simulink model "Modelsim"  (R2024a)
settings: Solver=VariableStepAuto  StartTime=0.0  StopTime=60  RelTol=1e-3
PreLoadFcn:
  | maxNumErrs = 100;
  | maxNumBits = 1e6;
  | EbNo = 4;
undefined symbols (not defined in the file): designMultirateFIR, SimPara
libraries: commchan3 x3, simulink x2, commcnvcod2 x2, dspvision x2, commdigbbndpm3 x2, commfilt2 x2, dspindex x2, matrix_library x2, dspsnks4 x1, commsink2 x1, dspmlti4 x1, commutil2 x1
settings Model: MinMaxOverflowLogging=MinMaxAndOverflow  SimulationMode=accelerator  Creator=The MathWorks, Inc.  LastModifiedBy=fiona
settings SolverCC: AlgebraicLoopSolver=TrustRegion
settings DataIOCC: LimitDataPoints=on  SaveFormat=Array  SignalLogging=off  SaveTime=off  ReturnWorkspaceOutputs=off
settings OptimizationCC: DefaultParameterBehavior=Inlined  ReuseModelBlockBuffer=off  ExpressionDepthLimit=2147483647  LocalBlockOutputs=off  InitFltsAndDblsToZero=on  LifeSpan=1  EfficientTunableParamExpr=on
settings DebuggingCC: SaveWithParameterizedLinksMsg=none  SignalResolutionControl=TryResolveAllWithWarning  SolverPrmCheckMsg=warning  MultiTaskDSMMsg=warning  MultiTaskCondExecSysMsg=none  UnconnectedInputMsg=warning  UnconnectedOutputMsg=warning  UnconnectedLineMsg=warning  StateNameClashWarn=warning  SFUnexpectedBacktrackingDiag=warning  SFNoUnconditionalDefaultTransitionDiag=warning  SFExecutionAtInitializationDiag=none  ArithmeticOperatorsInVariantConditions=warning
settings HardwareCC: ProdBitPerInt=16  ProdBitPerPointer=32  ProdBitPerSizeT=16  ProdBitPerPtrDiffT=16  ProdLargestAtomicFloat=None  ProdIntDivRoundTo=Floor  ProdWordSize=16  ProdHWDeviceType=16-bit Generic  TargetBitPerPointer=64  TargetBitPerSizeT=64  TargetBitPerPtrDiffT=64  TargetLongLongMode=on  TargetIntDivRoundTo=Zero  TargetEndianess=LittleEndian  TargetWordSize=64  TargetHWDeviceType=MATLAB Host  ProdEqTarget=off
settings ModelReferenceCC: EnableRefExpFcnMdlSchedulingChecks=on  PropagateSignalLabelsOutOfModel=off
settings SFSimCC: SimUseLocalCustomCode=off  MATLABDynamicMemAlloc=off  CustomCodeUndefinedFunction=UseInterfaceOnly
settings RTWCC: Description=Real-Time Workshop Embedded Coder (no auto configuration)  SystemTargetFile=ert.tlc  TemplateMakefile=ert_default_tmf  GenerateReport=on  RetainRTWFile=on  RTWUseLocalCustomCode=off  IncludeHyperlinkInReport=on  LaunchReport=on  GPUComputeCapability=3.5
settings CodeAppCC: CustomSymbolStrType=$N$R$M  StateflowObjectComments=on  InternalIdentifier=Classic
settings ERTTargetCC: TargetFcnLib=ansi_tfl_tmw.mat  MultiwordLength=2048  GenerateSampleERTMain=on  SupportAbsoluteTime=off  MatFileLogging=on  InlinedParameterPlacement=NonHierarchical  ERTCustomFileTemplate=example_file_process.tlc  ConvertIfToSwitch=off  SuppressUnreachableDefaultCases=off
settings ConfigComp: CovMetricSettings=dw  CovSaveCumulativeToWorkspaceVar=on  CovSaveSingleToWorkspaceVar=on  CovExternalEMLEnable=off

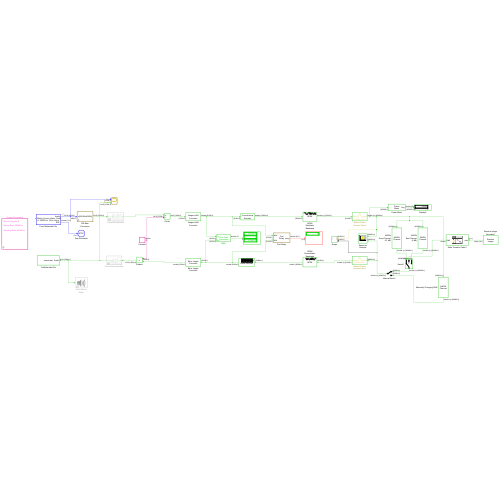
[thumbnail: Simulink's stored preview of the top-level diagram]
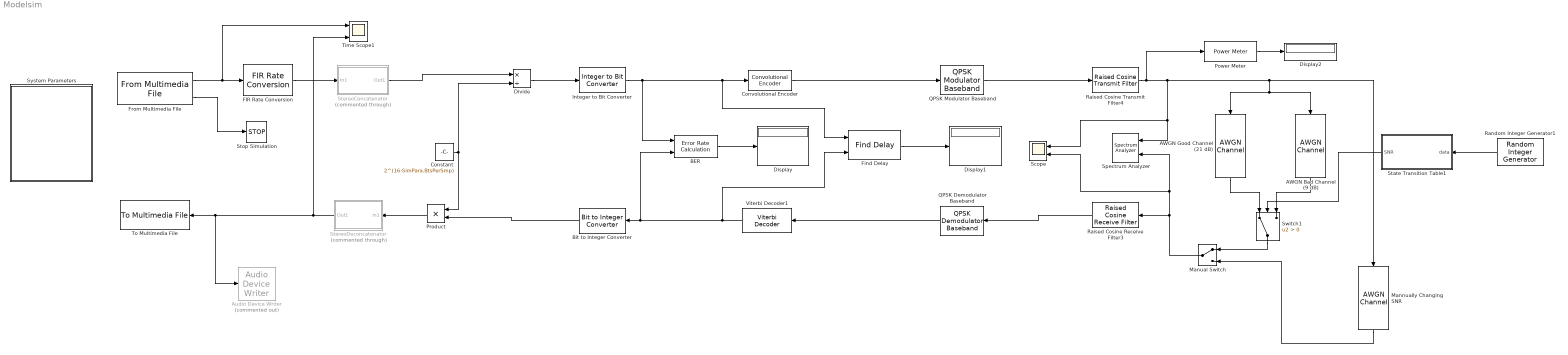
== system Modelsim ==
  AWGN Bad Channel (9 dB) : commchan3/AWGN Channel  LegacyMode=on  NoiseMethod="Signal to noise ratio  (SNR)"  noiseMode="Signal to noise ratio  (SNR)"  EbNo=10  EsNo=10  SNR=9  BitsPerSymbol=1  SignalPower=1  SamplesPerSymbol=1  SymbolPeriod=1  VarianceSource=Parameter  Variance=1  RandomStream=Global stream  Seed=67  SimulateUsing=Code generation
  AWGN Good Channel (21 dB) : commchan3/AWGN Channel  LegacyMode=on  NoiseMethod="Signal to noise ratio  (SNR)"  noiseMode="Signal to noise ratio  (SNR)"  EbNo=10  EsNo=10  SNR=21  BitsPerSymbol=1  SignalPower=1  SamplesPerSymbol=1  SymbolPeriod=1  VarianceSource=Parameter  Variance=1  RandomStream=Global stream  Seed=67  SimulateUsing=Code generation
  Audio Device Writer : dspsnks4/Audio Device Writer  Commented=on  Driver=DirectSound  Device=Default  InheritSampleRate=on  SampleRate=44100  BitDepth=16-bit integer  BufferSize=4096  NumBuffers=10  DefaultOutputChannelMapping=on  OutputChannelMapping=1:2  OutputNumUnderrunSamples=off  DriverIdx=1  DeviceWarnFlag=''
  BER : commsink2/Error Rate Calculation  N=20  st_delay=0  cp_mode=Entire frame  subframe=[]  PMode=Port  WsName=ErrorVec  RsMode2=off  stop=off  numErr=100  maxBits=1e7
  Bit to Integer Converter : simulink/Logic and Bit Operations/Bit to Integer Converter  nbits=SimPara.BtsPerSmp  bitOrder=MSB first  signedOutputValues=Signed  outDtype=Inherit via internal rule  outDtypeSigned=Inherit via internal rule
  Constant : Constant  Value=2^(16-SimPara.BtsPerSmp)
  Convolutional Encoder : commcnvcod2/Convolutional Encoder  trellis=poly2trellis(3, [7 5])  opMode=Continuous  DelayedResetAction=off  hasIniStPort=off  hasFinStPort=off  usePuncVector=off  punctureVector=[1; 1; 0; 1; 0; 1]  reset=Unused parameter value
  Display : Display
  Display1 : Display
  Display2 : Display
  Divide : Product  Inputs=*/  OutDataTypeStr=Inherit: Same as first input
  FIR Rate Conversion : dspmlti4/FIR Rate Conversion  FilterSource=Auto  L=SimPara.SmpRte  h=designMultirateFIR(3,2)  M=SimPara.SrcRte  FilterObject=FRC  rateMode=Allow multirate processing  AllowArbitraryInputLength=on  roundingMode=Floor  overflowMode=off  firstCoeffDataTypeStr=Inherit: Same word length as input  firstCoeffMin=[]  firstCoeffMax=[]  firstCoeffLastDataTypeStr=Inherit: Same word length as input  outputMin=[]  outputMax=[]
  Find Delay : commutil2/Find Delay  corrLength=1000  chgSigOP=off  stopUpdate=off  numConstDelay=3
  From Multimedia File : dspvision/From Multimedia File  inputFilename=C:\UBC\ELEC391\SoundFiles\Mono_16bit_22kHz_Uncom_60sec_PinkPanther.wav  readRange=[1 Inf]  loop=on  numPlays=1  outputStreams=Audio only  videoDataType=single  audioDataType=int16  inheritSampleTime=on  userDefinedSampleTime=1/30  noAudioOutput=off  isIntensityVideo=off  fourcc=RGB  colorVideoFormat=Separate color signals  outputEOF=on  dataOrg=Column-major  audioFrameSize=1024  computeAudioFrameSize=off  outSamplingMode=Sample based
      settings: LibrarySourceBlock=audiosources/From Multimedia File
  Integer to Bit Converter : simulink/Logic and Bit Operations/Integer to Bit Converter  nbits=SimPara.BtsPerSmp  signedInputValues=Signed  bitOrder=MSB first  outDtype=double
  Mannually Changing SNR : commchan3/AWGN Channel  LegacyMode=off  NoiseMethod="Signal to noise ratio  (SNR)"  noiseMode="Signal to noise ratio  (SNR)"  EbNo=10  EsNo=10  SNR=10  BitsPerSymbol=1  SignalPower=1  SamplesPerSymbol=1  SymbolPeriod=1  VarianceSource=Parameter  Variance=1  RandomStream=Global stream  Seed=67  SimulateUsing=Code generation
  Manual Switch : ManualSwitch
  Power Meter : dspstat3/Power Meter  Measurement=Average power  ReferenceLoad=1  OutputPowerUnits=Watts  WindowLength=256  OverlapLength=255  AllowArbitraryInputLength=off  ComputeCCDF=off  PowerRange=50  PowerResolution=0.1  CCDFOutput=Relative power (dB above average power)  ProbabilityVector=[ 10; 1; 0.1; 0.01; 0.001; 0.0001 ]  RelativePowerVector=[ 0; 3; 6; 9; 12 ]  ResetPort=off  SimulateUsing=Interpreted execution
  Product : Product  OutDataTypeStr=int16
  QPSK Demodulator Baseband : commdigbbndpm3/QPSK Demodulator Baseband  OutType=Bit  DecType=Hard decision  VarSource=Dialog  Variance=1  Dec=Binary  Ph=pi/4  outDtype1=Inherit via internal rule  outDtype2=Inherit via internal rule  derotateFactorWordLen=16  derotateFactorDataTypeStr=Inherit: Same word length as input  derotateFactorLastDataTypeStr=Inherit: Same word length as input
  QPSK Modulator Baseband : commdigbbndpm3/QPSK Modulator Baseband  InType=Bit  Enc=Binary  Ph=pi/4  outDtype=double  outWordLen=16  outUDDataType=sfix(16)  outFracLenMode=Best precision  outFracLen=15  outDataTypeStr=double  outLastDataTypeStr=double
  Raised Cosine Receive Filter3 : commfilt2/Raised Cosine Receive Filter  filtType=Square root  R=0.8  filtSpan=4  N=5  downFactor=5  downOffset=0  filterGain=1  InputProcessing=Columns as channels (frame based)  RateOptions=Enforce single-rate processing  framing=Mute  checkCoeff=on  variableName=rcRxFilt3  currentFiltSpan=10  D=5  inputOffset=0  sampMode=Mute  saveAsFlag=0  rateMode=Downsampling  checkGain=Normalized  launchFVT=on  roundingMode=Floor  overflowMode=off  coeffDataTypeStr=Inherit: Same word length as input  coeffMin=[]  coeffMax=[]  coeffLastDataTypeStr=Inherit: Same word length as input  accumDataTypeStr=Inherit: Same as product output  accumLastDataTypeStr=Inherit: Same as product output  outputDataTypeStr=Inherit: Same as accumulator  outputMin=[]  outputMax=[]  outputLastDataTypeStr=Inherit: Same as accumulator
      settings: LibrarySourceBlock=|
      | commhdlfilt/Raised Cosine
      | Receive Filter
  Raised Cosine Transmit Filter4 : commfilt2/Raised Cosine Transmit Filter  filtType=Square root  R=0.8  filtSpan=4  N=5  filterGain=1  InputProcessing=Columns as channels (frame based)  RateOptions=Enforce single-rate processing  framing=Mute  checkCoeff=on  variableName=rcTxFilt4  checkGain=Normalized  sampMode=Mute  saveAsFlag=0  currentFiltSpan=10  D=5  launchFVT=on  roundingMode=Floor  overflowMode=off  coeffDataTypeStr=Inherit: Same word length as input  coeffMin=[]  coeffMax=[]  coeffLastDataTypeStr=Inherit: Same word length as input  outputDataTypeStr=Inherit: Same as accumulator  outputMin=[]  outputMax=[]  outputLastDataTypeStr=Inherit: Same as accumulator
      settings: LibrarySourceBlock=|
      | commhdlfilt/Raised Cosine
      | Transmit Filter
  Random Integer Generator1 : commrandsrc3/Random Integer Generator  SetSize=100  SeedSource=Auto  Seed=0  SampleTime=0.0256  SamplesPerFrame=1  OutputDataType=single  SimulateUsing=Interpreted execution
  Scope : Scope  NumInputPorts=2
  Spectrum Analyzer : SpectrumAnalyzer  NumInputPorts=2  WindowPosition=[1.000000,49.000000,1504.000000,932.000000,]  ScopeFrameLocation=window  FrequencySpan=Start and stop frequencies  StartFrequency=0  StopFrequency=600000  YLimits=[-142.8961798129679,30.326241209565428]  ShowLegend=on  SelectedToolstripTab=spectrumAnalyzerToolstrip.channelMeasurementsTab  MeasurementChannel=2
  State Transition Table1 : State Transition Table  TreatAsAtomicUnit=on
  StereoConcatenator : Subsystem  Commented=through
  StereoDeconcatenator : Subsystem  Commented=through
  Stop Simulation : Stop
  Switch1 : Switch  Criteria=u2 > Threshold  SaturateOnIntegerOverflow=off  InputSameDT=off
  System Parameters : Subsystem  mask{BtsPerSmp=8, SrcRte=22050, SmpRte=40000}
      mask prompts: BtsPerSmp "BitsPerSample"; SrcRte "Source Rate (Hz)"; SmpRte "Sampling Rate (Hz)"
      mask init:
      | info.BtsPerSmp = BtsPerSmp;
      | info.SmpRte = SmpRte;
      | info.SrcRte = SrcRte;
      | 
      | assignin('base', 'SimPara', info);
      mask DialogControl SimVar Prompt: SimVariables
      mask Display:
      | text( ...
      |     10, 140, ...
      |     [ ...
      |     '\n\nBits Per Sample: ', num2str(BtsPerSmp), ...
      |     '\n\nSource Rate: ', num2str(SrcRte) ' Hz', ...
      |     '\n\nSampling Rate: ', num2str(SmpRte) ' Hz'], ...
      |     'horizontalAlignment', 'left' ...
      |     )
  Time Scope1 : Scope  NumInputPorts=3
  To Multimedia File : dspvision/To Multimedia File  outputFilename=C:\UBC\ELEC391\output.wav  streamSelection=Audio only  videoCompressor=None (uncompressed)  audioCompressor=None (uncompressed)  imagePorts=One multidimensional signal  fileType=WAV  audioDatatype=Determine from input data type  fourcc=RGB  audioBitRate=128  audioQuality=75  videoQuality=75  mj2000CompFactor=10
      settings: LibrarySourceBlock=audiosinks/To Multimedia File
  Viterbi Decoder1 : commcnvcod2/Viterbi Decoder  trellis=poly2trellis(3, [7 5])  isPunctured=off  punctureVector=[1; 1; 0; 1; 0; 1]  erasures=off  dectype=Hard decision  nsdecb=3  runSigValErrCheck=off  tbdepth=16  opmode=Continuous  reset=off  delayedResetAction=off  smWordLength=16  outDataType=double
  wires:
  BER/1 -> Display/1
  From Multimedia File/1 -> Time Scope1/1, FIR Rate Conversion/1
  FIR Rate Conversion/1 -> StereoConcatenator/1(In1)
  Divide/1 -> Integer to Bit Converter/1
  StereoDeconcatenator/1(Out1) -> Audio Device Writer/1, To Multimedia File/1, Time Scope1/3
  Product/1 -> StereoDeconcatenator/1(In1)
  StereoConcatenator/1(Out1) -> Divide/1
  Bit to Integer Converter/1 -> Product/2
  Constant/1 -> Product/1, Divide/2
  From Multimedia File/2 -> Stop Simulation/1
  QPSK Modulator Baseband/1 -> Raised Cosine Transmit Filter4/1
  QPSK Demodulator Baseband/1 -> Viterbi Decoder1/1
  Integer to Bit Converter/1 -> BER/1, Find Delay/1, Convolutional Encoder/1
  Raised Cosine Receive Filter3/1 -> QPSK Demodulator Baseband/1
  Convolutional Encoder/1 -> QPSK Modulator Baseband/1
  Random Integer Generator1/1 -> State Transition Table1/1(data)
  AWGN Good Channel (21 dB)/1 -> Switch1/1
  AWGN Bad Channel (9 dB)/1 -> Switch1/3
  State Transition Table1/1(SNR) -> Switch1/2
  Raised Cosine Transmit Filter4/1 -> Scope/1, Spectrum Analyzer/1, Mannually Changing SNR/1, AWGN Bad Channel (9 dB)/1, AWGN Good Channel (21 dB)/1, Power Meter/1
  Viterbi Decoder1/1 -> Find Delay/2, BER/2, Bit to Integer Converter/1
  Find Delay/1 -> Display1/1
  Power Meter/1 -> Display2/1
  Manual Switch/1 -> Scope/2, Spectrum Analyzer/2, Raised Cosine Receive Filter3/1
  Switch1/1 -> Manual Switch/1
  Mannually Changing SNR/1 -> Manual Switch/2

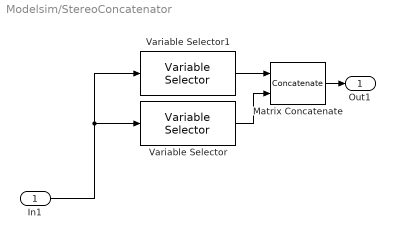
== system Modelsim/StereoConcatenator ==
  In1 : Inport
  Matrix Concatenate : Concatenate  ConcatenateDimension=2
  Variable Selector : dspindex/Variable Selector  NumInputs=1  rowsOrCols=Columns  IdxMode=Fixed  Elements=[1]  ZerOneIdxMode=One-based  errmode=Clip Index  FillMode=on  FillValues=0
  Variable Selector1 : dspindex/Variable Selector  NumInputs=1  rowsOrCols=Columns  IdxMode=Fixed  Elements=[2]  ZerOneIdxMode=One-based  errmode=Clip Index  FillMode=on  FillValues=0
  Out1 : Outport
  wires:
  Variable Selector1/1 -> Matrix Concatenate/1
  In1/1 -> Variable Selector1/1, Variable Selector/1
  Variable Selector/1 -> Matrix Concatenate/2
  Matrix Concatenate/1 -> Out1/1

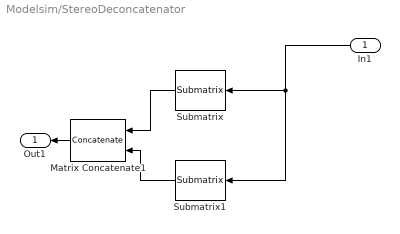
== system Modelsim/StereoDeconcatenator ==
  In1 : Inport
  Matrix Concatenate1 : Concatenate  Mode=Multidimensional array  ConcatenateDimension=2
  Submatrix : matrix_library/Submatrix  RowSpan=Range of rows  RowStartMode=First  RowStartIndex=1  RowEndMode=Offset from middle  RowEndIndex=-1  ColSpan=All columns  ColStartMode=First  ColStartIndex=1  ColEndMode=Last  ColEndIndex=1
  Submatrix1 : matrix_library/Submatrix  RowSpan=Range of rows  RowStartMode=Middle  RowStartIndex=1  RowEndMode=Last  RowEndIndex=-1  ColSpan=All columns  ColStartMode=First  ColStartIndex=1  ColEndMode=Last  ColEndIndex=1
  Out1 : Outport
  wires:
  Matrix Concatenate1/1 -> Out1/1
  In1/1 -> Submatrix1/1, Submatrix/1
  Submatrix1/1 -> Matrix Concatenate1/2
  Submatrix/1 -> Matrix Concatenate1/1

== system Modelsim/System Parameters ==

== stateflow chart Modelsim/State Transition Table1 ==
  state state1_G_
  state state2_B_
  (default) -> state1_G_
  state1_G_ -> (junction 21) [order 2] : {SNR = 1}
  (junction 21) -> state1_G_
  state1_G_ -> state2_B_ [order 1] : [data < 3]
      | {SNR = 1}
  state2_B_ -> state1_G_ [order 1] : [data < 25]
      | {SNR = -1}
  state2_B_ -> (junction 26) [order 2] : {SNR = -1}
  (junction 26) -> state2_B_
  data: data input; SNR output
